simulink model "dx_hand_model_rai3"  (R2017b)
settings: Solver=ode3  StartTime=0.0  StopTime=inf  FixedStep=0.01  RelTol=1e-3  EnableMultiTasking=on
InitFcn:
  | cutFreq = 0.1; % T
  | sampleTime = 0.01;
  | filt = tf(1,[cutFreq 1]);
  | filt = c2d(filt,sampleTime);
  | 
  | cutFreq2 = 1;
  | filt2 = tf(1,[cutFreq2 1]);
  | filt2 = c2d(filt2,sampleTime);
  | 
  | update_param = 2;
  | 
  | ampliFactor = 1.60;
  | ampliFactorMiddle = 2.00;
  | ampliFactorDistal = 1;
  | 
  | % Set Hand Address
  | RightHandAddress = '10.24.4.91';
  | Verosim = '10.100.39.22'
  | LeftHandAddress = '10.24.4.90'
  | 
  | max_force = 12; % Newton
model workspace (MAT data in the model file):
  SL_ROS_VariableLengthArrays_MaxSizes : struct (value not decoded)
libraries: robotlib x134, simulink_extras x28, simulink x16, dspnetwork x5, etargetslib x4
(part 17 of 19)

== matlab function dx_hand_model_rai3/Thumb/Proximal and Distal Phalanx/Teorema Coseni ==
  data: MCP input; PIP_FE output; PIP input; K input
function PIP_FE = fcn(MCP,PIP,K)
K_MCP_2 = (MCP(1) - K(1))^2 + (MCP(2) - K(2))^2 + (MCP(3) - K(3))^2;
K_PIP_2 = (PIP(1) - K(1))^2 + (PIP(2) - K(2))^2 + (PIP(3) - K(3))^2;
PIP_MCP_2 = (PIP(1) - MCP(1))^2 + (PIP(2) - MCP(2))^2 + (PIP(3) - MCP(3))^2;

PIP_FE_temp = pi- acos( complex((- K_MCP_2 + K_PIP_2 + PIP_MCP_2) / (2 * sqrt( K_PIP_2 * PIP_MCP_2 )) )); 

PIP_FE = PIP_FE_temp;

== matlab function dx_hand_model_rai3/Thumb/Proximal and Distal Phalanx/Get Min ==
  data: x output; x_in input; y output; z output; y_in input; z_in input
function [x,y,z] = get_min(x_in,y_in,z_in)
[val, where] = min(z_in);
x = x_in(where);
y = y_in(where);
z = z_in(where);

== matlab function dx_hand_model_rai3/Ring Finger /Position-Force Architecture/Optimized_Static_Problem ==
  data: Jcomponents input; y output; force_vector input
function y = fcn(Jcomponents, force_vector)
% Utilizzo la rendering strategy in the Force Space proposta da Mine
j_f = [0;0];
j_f = [force_vector(1);force_vector(2)];

Ja = [single(Jcomponents(1)); single(Jcomponents(3))];
Jp = [single(Jcomponents(2)); single(Jcomponents(4))];

% J = [Ja Jp];

a_f = Ja'*(eye(2)-Jp*inv(Jp'*Jp)*Jp')*j_f;

y = a_f;

== matlab function dx_hand_model_rai3/Ring Finger /Position-Position/Classic_Static_Problem ==
  data: Jcomponents input; rate output; operational_space input
function rate = fcn(Jcomponents, operational_space)
% Utilizzo la rendering strategy in the Force Space proposta da Mine
j_f = [operational_space(1);operational_space(2)];

Ja = [single(Jcomponents(1)); single(Jcomponents(3))];
Jp = [single(Jcomponents(2)); single(Jcomponents(4))];

% J = [Ja Jp];

a_f = Ja'*j_f;

rate = a_f;

== matlab function dx_hand_model_rai3/Ring Finger /Position-Position/Optimized_Static_Problem ==
  data: Jcomponents input; y output; force_vector input
function y = fcn(Jcomponents, force_vector)
% Utilizzo la rendering strategy in the Force Space proposta da Mine
j_f = [0;0];
j_f = [force_vector(1);force_vector(2)];

Ja = [single(Jcomponents(1)); single(Jcomponents(3))];
Jp = [single(Jcomponents(2)); single(Jcomponents(4))];

% J = [Ja Jp];

a_f = Ja'*(eye(2)-Jp*inv(Jp'*Jp)*Jp')*j_f;

y = a_f;

== matlab function dx_hand_model_rai3/Ring Finger /Pre-Proc/IsNan  ==
  data: Jin input; J output; J_k1 input
function J = fcn(Jin, J_k1)
% Utilizzo la rendering strategy in the Force Space proposta da 
J = single(zeros(1,4));
for i=1:4
    if isinf(Jin(i)) || isnan(Jin(i))
        Jin(i) = J_k1(i);
    end
    J(i) = Jin(i);
end
